simulink model "lock_srw_vB_windows"  (R2020a)
settings: Solver=FixedStepAuto  StartTime=0.0  StopTime=inf  RelTol=1e-3
model workspace (MAT data in the model file):
  PLC_IP_Address = 'localhost'
libraries: dspnetwork x29, simulink x2, utility x1
(part 1 of 2)
settings Model: SimulationMode=accelerator  EnablePacing=on  Creator=SueAnne  LastModifiedBy=jrsma
settings DataIOCC: ReturnWorkspaceOutputs=off
settings DebuggingCC: PregeneratedLibrarySubsystemCodeDiagnostic=none  ArithmeticOperatorsInVariantConditions=warning
settings SFSimCC: SimUseLocalCustomCode=off  CustomCodeUndefinedFunction=UseInterfaceOnly
settings RTWCC: PackageGeneratedCodeAndArtifacts=on  PackageName=Lock  RTWUseLocalCustomCode=off

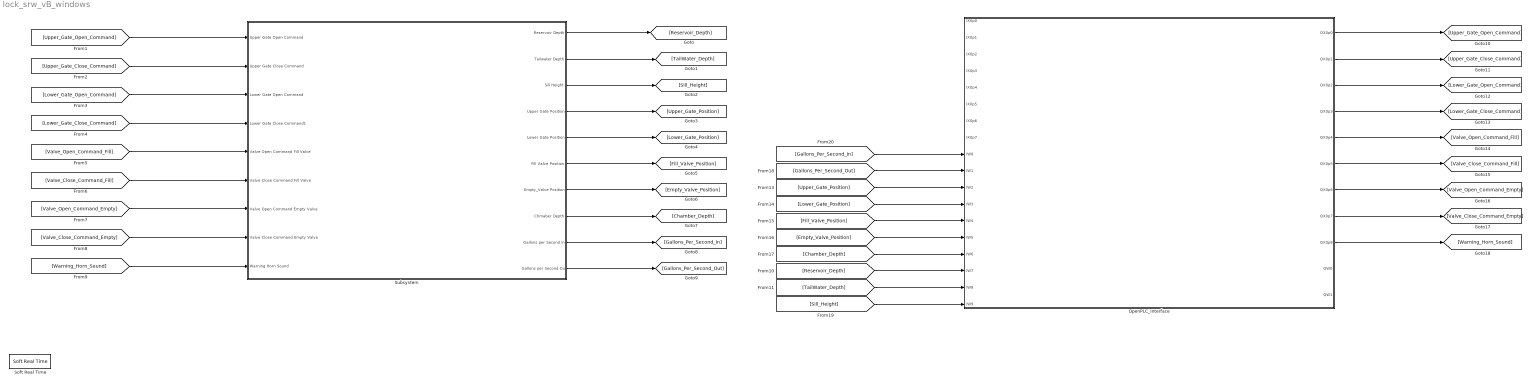
== system lock_srw_vB_windows ==
  OpenPLC_Interface : Subsystem
  Soft Real Time : utility/Soft Real Time  x=1
      settings: SourceProductName=Soft Real Time Lib
  Subsystem : Subsystem
  wires:
  [Upper_Gate_Open_Command] -> Subsystem/1(Upper Gate Open Command)
  [Upper_Gate_Close_Command] -> Subsystem/2(Upper Gate Close Command)
  [Lower_Gate_Open_Command] -> Subsystem/3(Lower Gate Open Command)
  [Lower_Gate_Close_Command] -> Subsystem/4(Lower Gate Close Command1)
  [Valve_Open_Command_Fill] -> Subsystem/5(Valve Open Command Fill Valve)
  [Valve_Close_Command_Fill] -> Subsystem/6(Valve Close Command Fill Valve)
  [Valve_Open_Command_Empty] -> Subsystem/7(Valve Open Command Empty Valve)
  [Valve_Close_Command_Empty] -> Subsystem/8(Valve Close Command Empty Valve)
  [Warning_Horn_Sound] -> Subsystem/9(Warning Horn Sound)
  Subsystem/1(Reservoir Depth) -> [Reservoir_Depth]
  Subsystem/2(Tailwater Depth) -> [TailWater_Depth]
  Subsystem/3(Sill Height) -> [Sill_Height]
  Subsystem/4(Upper Gate Position) -> [Upper_Gate_Position]
  Subsystem/5(Lower Gate Position) -> [Lower_Gate_Position]
  Subsystem/6(Fill Valve Position) -> [Fill_Valve_Position]
  Subsystem/7(Empty_Valve Position) -> [Empty_Valve_Position]
  Subsystem/8(Chmaber Depth) -> [Chamber_Depth]
  Subsystem/9(Gallons per Second In) -> [Gallons_Per_Second_In]
  Subsystem/10(Gallons per Second Ou) -> [Gallons_Per_Second_Out]
  [Sill_Height] -> OpenPLC_Interface/18(IW9)
  OpenPLC_Interface/1(QX0p0) -> [Upper_Gate_Open_Command]
  OpenPLC_Interface/2(QX0p1) -> [Upper_Gate_Close_Command]
  OpenPLC_Interface/3(QX0p2) -> [Lower_Gate_Open_Command]
  OpenPLC_Interface/4(QX0p3) -> [Lower_Gate_Close_Command]
  OpenPLC_Interface/5(QX0p4) -> [Valve_Open_Command_Fill]
  OpenPLC_Interface/6(QX0p5) -> [Valve_Close_Command_Fill]
  OpenPLC_Interface/7(QX0p6) -> [Valve_Open_Command_Empty]
  OpenPLC_Interface/8(QX0p7) -> [Valve_Close_Command_Empty]
  OpenPLC_Interface/9(QX0p8) -> [Warning_Horn_Sound]
  [Gallons_Per_Second_In] -> OpenPLC_Interface/9(IW0)
  [TailWater_Depth] -> OpenPLC_Interface/17(IW8)
  [Reservoir_Depth] -> OpenPLC_Interface/16(IW7)
  [Chamber_Depth] -> OpenPLC_Interface/15(IW6)
  [Empty_Valve_Position] -> OpenPLC_Interface/14(IW5)
  [Fill_Valve_Position] -> OpenPLC_Interface/13(IW4)
  [Lower_Gate_Position] -> OpenPLC_Interface/12(IW3)
  [Upper_Gate_Position] -> OpenPLC_Interface/11(IW2)
  [Gallons_Per_Second_Out] -> OpenPLC_Interface/10(IW1)

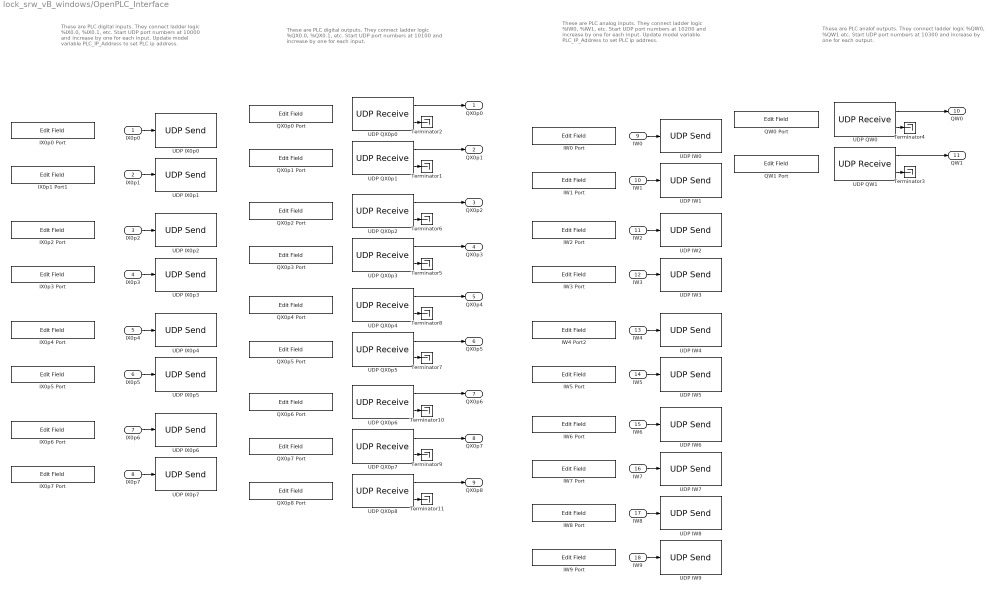
== system lock_srw_vB_windows/OpenPLC_Interface ==
  note: These are PLC digital inputs. They connect
      | ladder logic %IX0.0, %IX0.1, etc.
      |
      | Start UDP port numbers at 10000 and
      | increase by one for each input.
      |
      | Update model variable PLC_IP_Address
      | to set PLC ip address.
  note: These are PLC digital outputs. They connect
      | ladder logic %QX0.0, %QX0.1, etc.
      |
      | Start UDP port numbers at 10100 and increase
      | by one for each input.
  note: These are PLC analog inputs. They connect
      | ladder logic %IW0, %IW1, etc.
      |
      | Start UDP port numbers  at 10200 and
      | increase by one for each input.
      |
      | Update model variable PLC_IP_Address
      | to set PLC ip address.
  note: These are PLC analof outputs. They connect
      | ladder logic %QW0, %QW1 etc.
      |
      | Start UDP port numbers at 10300 and increase
      | by one for each output.
  "IX0p0 " : Inport
  IX0p1 : Inport  Port=2
  IX0p2 : Inport  Port=3
  IX0p3 : Inport  Port=4
  IX0p4 : Inport  Port=5
  IX0p5 : Inport  Port=6
  IX0p6 : Inport  Port=7
  IX0p7 : Inport  Port=8
  IW0 : Inport  Port=9
  IW1 : Inport  Port=10
  IW2 : Inport  Port=11
  IW3 : Inport  Port=12
  IW4 : Inport  Port=13
  IW5 : Inport  Port=14
  IW6 : Inport  Port=15
  IW7 : Inport  Port=16
  IW8 : Inport  Port=17
  IW9 : Inport  Port=18
  IW0 Port : EditField  LabelPosition=Hide  ShowInitialText=on  Alignment=Center
  IW1 Port : EditField  LabelPosition=Hide  ShowInitialText=on  Alignment=Center
  IW2 Port : EditField  LabelPosition=Hide  ShowInitialText=on  Alignment=Center
  IW3 Port : EditField  LabelPosition=Hide  ShowInitialText=on  Alignment=Center
  IW4 Port2 : EditField  LabelPosition=Hide  ShowInitialText=on  Alignment=Center
  IW5 Port : EditField  LabelPosition=Hide  ShowInitialText=on  Alignment=Center
  IW6 Port : EditField  LabelPosition=Hide  ShowInitialText=on  Alignment=Center
  IW7 Port : EditField  LabelPosition=Hide  ShowInitialText=on  Alignment=Center
  IW8 Port : EditField  LabelPosition=Hide  ShowInitialText=on  Alignment=Center
  IW9 Port : EditField  LabelPosition=Hide  ShowInitialText=on  Alignment=Center
  IX0p0 Port : EditField  LabelPosition=Hide  ShowInitialText=on  Alignment=Center
  IX0p1 Port1 : EditField  LabelPosition=Hide  ShowInitialText=on  Alignment=Center
  IX0p2 Port : EditField  LabelPosition=Hide  ShowInitialText=on  Alignment=Center
  IX0p3 Port : EditField  LabelPosition=Hide  ShowInitialText=on  Alignment=Center
  IX0p4 Port : EditField  LabelPosition=Hide  ShowInitialText=on  Alignment=Center
  IX0p5 Port : EditField  LabelPosition=Hide  ShowInitialText=on  Alignment=Center
  IX0p6 Port : EditField  LabelPosition=Hide  ShowInitialText=on  Alignment=Center
  IX0p7 Port : EditField  LabelPosition=Hide  ShowInitialText=on  Alignment=Center
  QW0 Port : EditField  LabelPosition=Hide  ShowInitialText=on  Alignment=Center
  QW1 Port : EditField  LabelPosition=Hide  ShowInitialText=on  Alignment=Center
  QX0p0 Port : EditField  LabelPosition=Hide  ShowInitialText=on  Alignment=Center
  QX0p1 Port : EditField  LabelPosition=Hide  ShowInitialText=on  Alignment=Center
  QX0p2 Port : EditField  LabelPosition=Hide  ShowInitialText=on  Alignment=Center
  QX0p3 Port : EditField  LabelPosition=Hide  ShowInitialText=on  Alignment=Center
  QX0p4 Port : EditField  LabelPosition=Hide  ShowInitialText=on  Alignment=Center
  QX0p5 Port : EditField  LabelPosition=Hide  ShowInitialText=on  Alignment=Center
  QX0p6 Port : EditField  LabelPosition=Hide  ShowInitialText=on  Alignment=Center
  QX0p7 Port : EditField  LabelPosition=Hide  ShowInitialText=on  Alignment=Center
  "QX0p8 Port " : EditField  LabelPosition=Hide  ShowInitialText=on  Alignment=Center
  Terminator{1..11} (11 alike) : Terminator
  UDP IW0 : dspnetwork/UDP Send  remoteURL='localhost'  remotePort=10200  localURL='255.255.255.255'  localPortSource=Automatically determine  localPort=-1  sendBufferSize=8192  sampletime=-1  blockPlatform=LINUX  separateLengthPort=0
  UDP IW1 : dspnetwork/UDP Send  remoteURL='localhost'  remotePort=10201  localURL='255.255.255.255'  localPortSource=Automatically determine  localPort=-1  sendBufferSize=8192  sampletime=-1  blockPlatform=LINUX  separateLengthPort=0
  UDP IW2 : dspnetwork/UDP Send  remoteURL='localhost'  remotePort=10202  localURL='255.255.255.255'  localPortSource=Automatically determine  localPort=-1  sendBufferSize=8192  sampletime=-1  blockPlatform=LINUX  separateLengthPort=0
  UDP IW3 : dspnetwork/UDP Send  remoteURL='localhost'  remotePort=10203  localURL='255.255.255.255'  localPortSource=Automatically determine  localPort=-1  sendBufferSize=8192  sampletime=-1  blockPlatform=LINUX  separateLengthPort=0
  UDP IW4 : dspnetwork/UDP Send  remoteURL='localhost'  remotePort=10204  localURL='255.255.255.255'  localPortSource=Automatically determine  localPort=-1  sendBufferSize=8192  sampletime=-1  blockPlatform=LINUX  separateLengthPort=0
  UDP IW5 : dspnetwork/UDP Send  remoteURL='localhost'  remotePort=10205  localURL='255.255.255.255'  localPortSource=Automatically determine  localPort=-1  sendBufferSize=8192  sampletime=-1  blockPlatform=LINUX  separateLengthPort=0
  UDP IW6 : dspnetwork/UDP Send  remoteURL='localhost'  remotePort=10206  localURL='255.255.255.255'  localPortSource=Automatically determine  localPort=-1  sendBufferSize=8192  sampletime=-1  blockPlatform=LINUX  separateLengthPort=0
  UDP IW7 : dspnetwork/UDP Send  remoteURL='localhost'  remotePort=10207  localURL='255.255.255.255'  localPortSource=Automatically determine  localPort=-1  sendBufferSize=8192  sampletime=-1  blockPlatform=LINUX  separateLengthPort=0
  UDP IW8 : dspnetwork/UDP Send  remoteURL='localhost'  remotePort=10208  localURL='255.255.255.255'  localPortSource=Automatically determine  localPort=-1  sendBufferSize=8192  sampletime=-1  blockPlatform=LINUX  separateLengthPort=0
  UDP IW9 : dspnetwork/UDP Send  remoteURL='localhost'  remotePort=10209  localURL='255.255.255.255'  localPortSource=Automatically determine  localPort=-1  sendBufferSize=8192  sampletime=-1  blockPlatform=LINUX  separateLengthPort=0
  UDP IX0p0 : dspnetwork/UDP Send  remoteURL='localhost'  remotePort=10000  localURL='255.255.255.255'  localPortSource=Automatically determine  localPort=-1  sendBufferSize=8192  sampletime=-1  blockPlatform=LINUX  separateLengthPort=0
  UDP IX0p1 : dspnetwork/UDP Send  remoteURL='localhost'  remotePort=10001  localURL='255.255.255.255'  localPortSource=Automatically determine  localPort=-1  sendBufferSize=8192  sampletime=-1  blockPlatform=LINUX  separateLengthPort=0
  UDP IX0p2 : dspnetwork/UDP Send  remoteURL='localhost'  remotePort=10002  localURL='255.255.255.255'  localPortSource=Automatically determine  localPort=-1  sendBufferSize=8192  sampletime=-1  blockPlatform=LINUX  separateLengthPort=0
  UDP IX0p3 : dspnetwork/UDP Send  remoteURL='localhost'  remotePort=10003  localURL='255.255.255.255'  localPortSource=Automatically determine  localPort=-1  sendBufferSize=8192  sampletime=-1  blockPlatform=LINUX  separateLengthPort=0
  UDP IX0p4 : dspnetwork/UDP Send  remoteURL='localhost'  remotePort=10004  localURL='255.255.255.255'  localPortSource=Automatically determine  localPort=-1  sendBufferSize=8192  sampletime=-1  blockPlatform=LINUX  separateLengthPort=0
  UDP IX0p5 : dspnetwork/UDP Send  remoteURL='localhost'  remotePort=10005  localURL='255.255.255.255'  localPortSource=Automatically determine  localPort=-1  sendBufferSize=8192  sampletime=-1  blockPlatform=LINUX  separateLengthPort=0
  UDP IX0p6 : dspnetwork/UDP Send  remoteURL='localhost'  remotePort=10006  localURL='255.255.255.255'  localPortSource=Automatically determine  localPort=-1  sendBufferSize=8192  sampletime=-1  blockPlatform=LINUX  separateLengthPort=0
  UDP IX0p7 : dspnetwork/UDP Send  remoteURL='localhost'  remotePort=10007  localURL='255.255.255.255'  localPortSource=Automatically determine  localPort=-1  sendBufferSize=8192  sampletime=-1  blockPlatform=LINUX  separateLengthPort=0
  UDP QW0 : dspnetwork/UDP Receive  localURL='0.0.0.0'  localPort=10300  remoteURL='0.0.0.0'  remotePort=-1  recvBufferSize=2  dims=1  signalDatatype=uint16  isComplex=off  isVarSize=off  showBlockingTime=on  blockingTime=0  sampletime=0.01  blockPlatform=LINUX
  UDP QW1 : dspnetwork/UDP Receive  localURL='0.0.0.0'  localPort=10301  remoteURL='0.0.0.0'  remotePort=-1  recvBufferSize=2  dims=1  signalDatatype=uint16  isComplex=off  isVarSize=off  showBlockingTime=on  blockingTime=0  sampletime=0.01  blockPlatform=LINUX
  UDP QX0p0 : dspnetwork/UDP Receive  localURL='0.0.0.0'  localPort=10100  remoteURL='0.0.0.0'  remotePort=-1  recvBufferSize=2  dims=1  signalDatatype=uint16  isComplex=off  isVarSize=off  showBlockingTime=on  blockingTime=0  sampletime=0.01  blockPlatform=LINUX
  UDP QX0p1 : dspnetwork/UDP Receive  localURL='0.0.0.0'  localPort=10101  remoteURL='0.0.0.0'  remotePort=-1  recvBufferSize=2  dims=1  signalDatatype=uint16  isComplex=off  isVarSize=off  showBlockingTime=on  blockingTime=0  sampletime=0.01  blockPlatform=LINUX
  UDP QX0p2 : dspnetwork/UDP Receive  localURL='0.0.0.0'  localPort=10102  remoteURL='0.0.0.0'  remotePort=-1  recvBufferSize=2  dims=1  signalDatatype=uint16  isComplex=off  isVarSize=off  showBlockingTime=on  blockingTime=0  sampletime=0.01  blockPlatform=LINUX
  UDP QX0p3 : dspnetwork/UDP Receive  localURL='0.0.0.0'  localPort=10103  remoteURL='0.0.0.0'  remotePort=-1  recvBufferSize=2  dims=1  signalDatatype=uint16  isComplex=off  isVarSize=off  showBlockingTime=on  blockingTime=0  sampletime=0.01  blockPlatform=LINUX
  UDP QX0p4 : dspnetwork/UDP Receive  localURL='0.0.0.0'  localPort=10104  remoteURL='0.0.0.0'  remotePort=-1  recvBufferSize=2  dims=1  signalDatatype=uint16  isComplex=off  isVarSize=off  showBlockingTime=on  blockingTime=0  sampletime=0.01  blockPlatform=LINUX
  UDP QX0p5 : dspnetwork/UDP Receive  localURL='0.0.0.0'  localPort=10105  remoteURL='0.0.0.0'  remotePort=-1  recvBufferSize=2  dims=1  signalDatatype=uint16  isComplex=off  isVarSize=off  showBlockingTime=on  blockingTime=0  sampletime=0.01  blockPlatform=LINUX
  UDP QX0p6 : dspnetwork/UDP Receive  localURL='0.0.0.0'  localPort=10106  remoteURL='0.0.0.0'  remotePort=-1  recvBufferSize=2  dims=1  signalDatatype=uint16  isComplex=off  isVarSize=off  showBlockingTime=on  blockingTime=0  sampletime=0.01  blockPlatform=LINUX
  UDP QX0p7 : dspnetwork/UDP Receive  localURL='0.0.0.0'  localPort=10107  remoteURL='0.0.0.0'  remotePort=-1  recvBufferSize=2  dims=1  signalDatatype=uint16  isComplex=off  isVarSize=off  showBlockingTime=on  blockingTime=0  sampletime=0.01  blockPlatform=LINUX
  UDP QX0p8 : dspnetwork/UDP Receive  localURL='0.0.0.0'  localPort=10108  remoteURL='0.0.0.0'  remotePort=-1  recvBufferSize=2  dims=1  signalDatatype=uint16  isComplex=off  isVarSize=off  showBlockingTime=on  blockingTime=0  sampletime=0.01  blockPlatform=LINUX
  QX0p0 : Outport
  QX0p1 : Outport  Port=2
  QX0p2 : Outport  Port=3
  QX0p3 : Outport  Port=4
  QX0p4 : Outport  Port=5
  QX0p5 : Outport  Port=6
  QX0p6 : Outport  Port=7
  QX0p7 : Outport  Port=8
  QX0p8 : Outport  Port=9
  QW0 : Outport  Port=10
  QW1 : Outport  Port=11
  wires:
  IX0p1/1 -> UDP IX0p1/1
  "IX0p0 "/1 -> UDP IX0p0/1
  UDP QX0p0/1 -> QX0p0/1
  UDP QX0p0/2 -> Terminator2/1
  UDP QX0p1/2 -> Terminator1/1
  UDP QX0p1/1 -> QX0p1/1
  IW1/1 -> UDP IW1/1
  IW0/1 -> UDP IW0/1
  UDP QW1/1 -> QW1/1
  UDP QW1/2 -> Terminator3/1
  UDP QW0/2 -> Terminator4/1
  UDP QW0/1 -> QW0/1
  IX0p2/1 -> UDP IX0p2/1
  IX0p3/1 -> UDP IX0p3/1
  IX0p7/1 -> UDP IX0p7/1
  IX0p6/1 -> UDP IX0p6/1
  IX0p4/1 -> UDP IX0p4/1
  IX0p5/1 -> UDP IX0p5/1
  UDP QX0p2/1 -> QX0p2/1
  UDP QX0p2/2 -> Terminator6/1
  UDP QX0p3/1 -> QX0p3/1
  UDP QX0p3/2 -> Terminator5/1
  UDP QX0p7/2 -> Terminator9/1
  UDP QX0p7/1 -> QX0p7/1
  UDP QX0p6/1 -> QX0p6/1
  UDP QX0p6/2 -> Terminator10/1
  UDP QX0p4/1 -> QX0p4/1
  UDP QX0p4/2 -> Terminator8/1
  UDP QX0p5/1 -> QX0p5/1
  UDP QX0p5/2 -> Terminator7/1
  IW3/1 -> UDP IW3/1
  IW2/1 -> UDP IW2/1
  IW7/1 -> UDP IW7/1
  IW5/1 -> UDP IW5/1
  IW4/1 -> UDP IW4/1
  IW6/1 -> UDP IW6/1
  IW9/1 -> UDP IW9/1
  IW8/1 -> UDP IW8/1
  UDP QX0p8/2 -> Terminator11/1
  UDP QX0p8/1 -> QX0p8/1

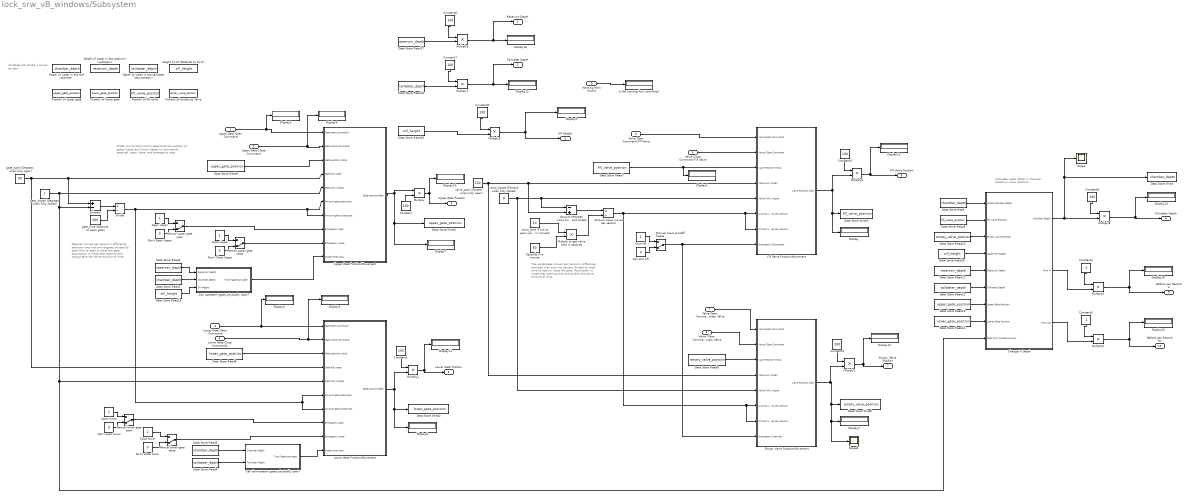
== system lock_srw_vB_windows/Subsystem ==
  note: These two function blocks determine the position of gates (upper and lower) based on commands received: open, close, and emergency stop.
  note: Variables are stored in boxes at right.
  note: Calculate water depth in chamber based on valve positions.
  note: Degrees moved per second is difference between max and min degrees divided by total time to open or close the gate. Assumption is made that opening and closing take the same amount of time.
  note: The percentage moved per second is difference between max and min percent divided by total time to open or close the gate. Assumption is made that opening and closing take the same amount of time.
  Upper Gate Open Command : Inport
  Upper Gate Close Command : Inport  Port=2
  Lower Gate Open Command : Inport  Port=3
  Lower Gate Close Command1 : Inport  Port=4
  Valve Open Command Fill Valve : Inport  Port=5
  Valve Close Command Fill Valve : Inport  Port=6
  Valve Open Command Empty Valve : Inport  Port=7
  Valve Close Command Empty Valve : Inport  Port=8
  Warning Horn Sound : Inport  Port=9
  Amount between valve fully open and closed : Sum  Inputs=-+  OutDataTypeStr=uint8
  Amount valve moves per second : Product  Inputs=*/  OutDataTypeStr=double
  Can downstream gates physically open? : Subsystem
  Can upstream gates physically open? : Subsystem
  Change in Depth : Subsystem
  Close Upper : Constant
  Close lower : Constant
  Constant{,1..3,6..9} (8 alike) : Constant  Value=100
  Constant4 : Constant  Value=.1
  Constant5 : Constant  Value=.1
  Data Store Read : DataStoreRead  DataStoreName=chamber_depth
  Data Store Read1 : DataStoreRead  Priority=0  DataStoreName=chamber_depth
  Data Store Read10 : DataStoreRead  DataStoreName=empty_valve_position
  Data Store Read11 : DataStoreRead  DataStoreName=reservoir_depth
  Data Store Read12 : DataStoreRead  DataStoreName=tailwater_depth
  Data Store Read13 : DataStoreRead  DataStoreName=upper_gate_position
  Data Store Read14 : DataStoreRead  DataStoreName=lower_gate_position
  Data Store Read15 : DataStoreRead  Priority=0  DataStoreName=sill_height
  Data Store Read16 : DataStoreRead  Priority=0  DataStoreName=sill_height
  Data Store Read17 : DataStoreRead  Priority=0  DataStoreName=reservoir_depth
  Data Store Read18 : DataStoreRead  Priority=0  DataStoreName=tailwater_depth
  Data Store Read19 : DataStoreRead  Priority=0  DataStoreName=sill_height
  Data Store Read2 : DataStoreRead  Priority=0  DataStoreName=reservoir_depth
  Data Store Read3 : DataStoreRead  DataStoreName=chamber_depth
  Data Store Read4 : DataStoreRead  DataStoreName=tailwater_depth
  Data Store Read5 : DataStoreRead  Priority=0  DataStoreName=upper_gate_position
  Data Store Read6 : DataStoreRead  Priority=0  DataStoreName=lower_gate_position
  Data Store Read7 : DataStoreRead  Priority=0  DataStoreName=fill_valve_position
  Data Store Read8 : DataStoreRead  Priority=0  DataStoreName=empty_valve_position
  Data Store Read9 : DataStoreRead  DataStoreName=fill_valve_position
  Data Store Write : DataStoreWrite  DataStoreName=chamber_depth
  Data Store Write1 : DataStoreWrite  Priority=9  DataStoreName=upper_gate_position
  Data Store Write2 : DataStoreWrite  Priority=9  DataStoreName=lower_gate_position
  Data Store Write3 : DataStoreWrite  Priority=9  DataStoreName=fill_valve_position
  Data Store Write4 : DataStoreWrite  Priority=9  DataStoreName=empty_valve_position
  Depth of water in the lock chamber : DataStoreMemory  DataStoreName=chamber_depth  ReadBeforeWriteMsg=warning  WriteAfterWriteMsg=warning  WriteAfterReadMsg=warning  InitialValue=42.5  ShowAdditionalParam=off
  Depth of water in the reservoir (upstream) : DataStoreMemory  DataStoreName=reservoir_depth  ReadBeforeWriteMsg=warning  WriteAfterWriteMsg=warning  WriteAfterReadMsg=warning  InitialValue=21  ShowAdditionalParam=off
  Depth of water in the tailwater (downstream) : DataStoreMemory  DataStoreName=tailwater_depth  ReadBeforeWriteMsg=warning  WriteAfterWriteMsg=warning  WriteAfterReadMsg=warning  InitialValue=21  ShowAdditionalParam=off
  Display{,1..16,18..19} (19 alike) : Display
  Divide : Product  Inputs=*/  OutDataTypeStr=double
  Don't Close Upper : Constant  Value=0
  Don't Open Upper : Constant  Value=0
  Don't close lower : Constant  Value=0
  Don't open lower : Constant  Value=0
  Empty Valve Position/Movement : Subsystem
  Fill Valve Position/Movement : Subsystem
  Height of sill (Defaults to 21.5') : DataStoreMemory  DataStoreName=sill_height  ReadBeforeWriteMsg=warning  WriteAfterWriteMsg=warning  WriteAfterReadMsg=warning  InitialValue=21.5  ShowAdditionalParam=off
  Is the warning horn sounding? : Display
  Lower Gate Position/Movement : Subsystem
  Manual lower gate close : ManualSwitch  CurrentSetting=0
  Manual lower gate open : ManualSwitch  CurrentSetting=0
  Manual upper gate close : ManualSwitch  CurrentSetting=0
  Manual upper gate open : ManualSwitch  CurrentSetting=0
  Manual valve shutoff/ freeze : ManualSwitch  CurrentSetting=0
  Multiply{,1..9} (10 alike) : Product
  Multiply to get valve time in seconds : Product  OutDataTypeStr=uint16
  Not shut off : Constant  Value=0  OutDataTypeStr=boolean
  Open Upper : Constant
  Open lower : Constant
  Position of emptying valve : DataStoreMemory  DataStoreName=empty_valve_position  ReadBeforeWriteMsg=warning  WriteAfterWriteMsg=warning  WriteAfterReadMsg=warning  ShowAdditionalParam=off
  Position of fill valve : DataStoreMemory  DataStoreName=fill_valve_position  ReadBeforeWriteMsg=warning  WriteAfterWriteMsg=warning  WriteAfterReadMsg=warning  ShowAdditionalParam=off  OutMin=0  OutMax=100  OutDataTypeStr=double
  Position of lower gate : DataStoreMemory  DataStoreName=lower_gate_position  ReadBeforeWriteMsg=warning  WriteAfterWriteMsg=warning  WriteAfterReadMsg=warning  InitialValue=7  ShowAdditionalParam=off
  Position of upper gate : DataStoreMemory  DataStoreName=upper_gate_position  ReadBeforeWriteMsg=warning  WriteAfterWriteMsg=warning  WriteAfterReadMsg=warning  InitialValue=7  ShowAdditionalParam=off
  Scope : Scope
  Scope1 : Scope
  Seconds in a minute : Constant  Value=60  OutDataTypeStr=uint8
  Shut off : Constant  OutDataTypeStr=boolean
  Subtract : Sum  Inputs=+-
  Upper Gate Position/Movement : Subsystem
  gate_closed (Degrees when fully closed) : Constant  Value=7
  gate_open (Degrees when fully open) : Constant  Value=90
  gate_time (Seconds to open gate) : Constant  Value=300
  valve_closed (Percent when fully closed) : Constant  Value=0  OutDataTypeStr=uint8
  valve_open (Percent when fully open) : Constant  Value=100  OutDataTypeStr=uint8
  "valve_time (Time to open valve, in minutes)" : Constant  Value=10  OutDataTypeStr=uint8
  Reservoir Depth : Outport
  Tailwater Depth : Outport  Port=2
  Sill Height : Outport  Port=3
  Upper Gate Position : Outport  Port=4
  Lower Gate Position : Outport  Port=5
  Fill Valve Position : Outport  Port=6
  Empty_Valve Position : Outport  Port=7
  Chmaber Depth : Outport  Port=8
  Gallons per Second In : Outport  Port=9
  Gallons per Second Ou : Outport  Port=10
  wires:
  Divide/1 -> Lower Gate Position/Movement/7(Amount gate closes/sec), Lower Gate Position/Movement/6(Amount gate opens/sec), Upper Gate Position/Movement/7(Amount gate closes/sec), Upper Gate Position/Movement/6(Amount gate opens/sec)
  Empty Valve Position/Movement/1(Valve Position After) -> Multiply2/2, Scope1/1, Display2/1, Data Store Write4/1
  Data Store Read1/1 -> Can upstream gates physically open?/2(Chamber Depth)
  Amount between valve fully open and closed/1 -> Amount valve moves per second/1
  Data Store Read3/1 -> Can downstream gates physically open?/1(Chamber Depth)
  Upper Gate Position/Movement/1(Gate position after) -> Multiply/1, Display7/1, Data Store Write1/1
  Constant3/1 -> Multiply3/1
  Fill Valve Position/Movement/1(Valve Position After) -> Multiply3/2, Data Store Write3/1, Display/1
  gate_closed (Degrees when fully closed)/1 -> Change in Depth/9(Gate Fully Closed Amount), Lower Gate Position/Movement/5(Gate fully closed), Subtract/2, Upper Gate Position/Movement/5(Gate fully closed)
  Lower Gate Position/Movement/1(Gate position after) -> Multiply1/2, Data Store Write2/1, Display8/1
  Manual lower gate open/1 -> Lower Gate Position/Movement/8(Emergency open)
  Can upstream gates physically open?/1(True if gate can open) -> Upper Gate Position/Movement/10(Water level okay)
  gate_time (Seconds to open gate)/1 -> Divide/2
  Can downstream gates physically open?/1(True if gate can open) -> Lower Gate Position/Movement/10(Water level okay)
  Amount valve moves per second/1 -> Fill Valve Position/Movement/7(Amount valve closes per second), Fill Valve Position/Movement/6(Amount valve opens per second), Empty Valve Position/Movement/7(Amount valve closes per second), Empty Valve Position/Movement/6(Amount valve opens per second)
  Data Store Read4/1 -> Can downstream gates physically open?/2(Tailwater Depth)
  Data Store Read6/1 -> Lower Gate Position/Movement/3(Gate position initial)
  Shut off/1 -> Manual valve shutoff/ freeze/1
  valve_closed (Percent when fully closed)/1 -> Fill Valve Position/Movement/5(Valve Fully Closed), Amount between valve fully open and closed/1, Empty Valve Position/Movement/5(Valve Fully Closed)
  Open lower/1 -> Manual lower gate open/1
  Data Store Read/1 -> Change in Depth/1(Initial Chamber Depth)
  Constant2/1 -> Multiply2/1
  Change in Depth/1(Chamber Depth) -> Multiply8/2, Scope/1, Data Store Write/1
  Don't Close Upper/1 -> Manual upper gate close/2
  Data Store Read11/1 -> Change in Depth/5(Reservoir Depth)
  Data Store Read9/1 -> Change in Depth/2(Fill Valve Position)
  Data Store Read17/1 -> Multiply6/2
  Data Store Read13/1 -> Change in Depth/7(Upper Gate Position)
  Data Store Read15/1 -> Can upstream gates physically open?/3(Sill Height)
  Change in Depth/3(Flow out) -> Multiply5/2
  gate_open (Degrees when fully open)/1 -> Lower Gate Position/Movement/4(Gate fully open), Subtract/1, Upper Gate Position/Movement/4(Gate fully open)
  Upper Gate Close Command/1 -> Upper Gate Position/Movement/2(Gate close command), Display4/1
  valve_open (Percent when fully open)/1 -> Amount between valve fully open and closed/2, Fill Valve Position/Movement/4(Valve Fully Open), Empty Valve Position/Movement/4(Valve Fully Open)
  Data Store Read7/1 -> Display1/1, Fill Valve Position/Movement/3(Valve Position Initial)
  Close lower/1 -> Manual lower gate close/1
  Manual valve shutoff/ freeze/1 -> Fill Valve Position/Movement/8(Emergency Disconnect), Empty Valve Position/Movement/8(Emergency Override)
  Constant/1 -> Multiply/2
  Data Store Read2/1 -> Can upstream gates physically open?/1(Reservoir Depth)
  Constant1/1 -> Multiply1/1
  Manual upper gate close/1 -> Upper Gate Position/Movement/9(Emergency close)
  Data Store Read16/1 -> Change in Depth/4(Upper Sill Height)
  Lower Gate Close Command1/1 -> Lower Gate Position/Movement/2(Gate close command), Display6/1
  Close Upper/1 -> Manual upper gate close/1
  Don't close lower/1 -> Manual lower gate close/2
  Not shut off/1 -> Manual valve shutoff/ freeze/2
  Multiply5/1 -> Gallons per Second Ou/1, Display19/1
  Data Store Read12/1 -> Change in Depth/6(Tailwater Depth)
  Data Store Read8/1 -> Empty Valve Position/Movement/3(Valve Position Initial)
  Change in Depth/2(Flow in) -> Multiply4/2
  Constant4/1 -> Multiply4/1
  Warning Horn Sound/1 -> Is the warning horn sounding?/1
  Multiply/1 -> Upper Gate Position/1, Display10/1
  Data Store Read5/1 -> Upper Gate Position/Movement/3(Gate position initial)
  Open Upper/1 -> Manual upper gate open/1
  Constant6/1 -> Multiply6/1
  Multiply to get valve time in seconds/1 -> Amount valve moves per second/2
  Don't open lower/1 -> Manual lower gate open/2
  Multiply7/1 -> Tailwater Depth/1, Display15/1
  Don't Open Upper/1 -> Manual upper gate open/2
  Seconds in a minute/1 -> Multiply to get valve time in seconds/2
  Constant7/1 -> Multiply7/1
  Manual upper gate open/1 -> Upper Gate Position/Movement/8(Emergency open)
  Data Store Read18/1 -> Multiply7/2
  Constant8/1 -> Multiply8/1
  Data Store Read10/1 -> Change in Depth/3(Empty Valve Position)
  Manual lower gate close/1 -> Lower Gate Position/Movement/9(Emergency close)
  Constant5/1 -> Multiply5/1
  Data Store Read14/1 -> Change in Depth/8(Lower Gate Position)
  Lower Gate Open Command/1 -> Lower Gate Position/Movement/1(Gate open command), Display5/1
  "valve_time (Time to open valve, in minutes)"/1 -> Multiply to get valve time in seconds/1
  Subtract/1 -> Divide/1
  Upper Gate Open Command/1 -> Display3/1, Upper Gate Position/Movement/1(Gate open command)
  Valve Open Command Fill Valve/1 -> Fill Valve Position/Movement/1(Valve Open Command)
  Valve Close Command Fill Valve/1 -> Fill Valve Position/Movement/2(Valve Close Command)
  Valve Open Command Empty Valve/1 -> Empty Valve Position/Movement/1(Valve Open Command)
  Valve Close Command Empty Valve/1 -> Empty Valve Position/Movement/2(Valve Close Command)
  Multiply6/1 -> Reservoir Depth/1, Display16/1
  Multiply1/1 -> Lower Gate Position/1, Display11/1
  Multiply3/1 -> Fill Valve Position/1, Display13/1
  Multiply2/1 -> Empty_Valve Position/1, Display12/1
  Multiply8/1 -> Chmaber Depth/1, Display14/1
  Multiply4/1 -> Gallons per Second In/1, Display18/1
  Data Store Read19/1 -> Multiply9/2
  Multiply9/1 -> Display9/1, Sill Height/1
  Constant9/1 -> Multiply9/1

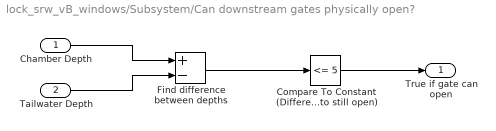
== system lock_srw_vB_windows/Subsystem/Can downstream gates physically open? ==
  Chamber Depth : Inport
  Tailwater Depth : Inport  Port=2
  Compare To Constant (Difference allowed between depths for gate to still open) : simulink/Logic and Bit Operations/Compare To Constant  relop=<=  const=5  OutDataTypeStr=boolean
  Find difference between depths : Sum  Inputs=+-
  True if gate can open : Outport  VectorParamsAs1DForOutWhenUnconnected=off
  wires:
  Chamber Depth/1 -> Find difference between depths/1
  Tailwater Depth/1 -> Find difference between depths/2
  Compare To Constant (Difference allowed between depths for gate to still open)/1 -> True if gate can open/1
  Find difference between depths/1 -> Compare To Constant (Difference allowed between depths for gate to still open)/1

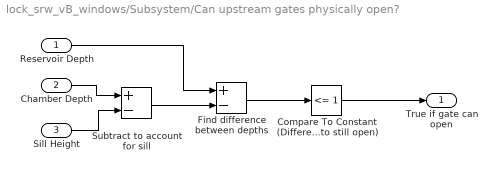
== system lock_srw_vB_windows/Subsystem/Can upstream gates physically open? ==
  Reservoir Depth : Inport
  Chamber Depth : Inport  Port=2
  Sill Height : Inport  Port=3
  Compare To Constant (Difference allowed between depths for gate to still open) : simulink/Logic and Bit Operations/Compare To Constant  relop=<=  const=1  OutDataTypeStr=boolean
  Find difference between depths : Sum  Inputs=+-
  Subtract to account for sill : Sum  Inputs=+-
  True if gate can open : Outport  VectorParamsAs1DForOutWhenUnconnected=off
  wires:
  Compare To Constant (Difference allowed between depths for gate to still open)/1 -> True if gate can open/1
  Find difference between depths/1 -> Compare To Constant (Difference allowed between depths for gate to still open)/1
  Subtract to account for sill/1 -> Find difference between depths/2
  Chamber Depth/1 -> Subtract to account for sill/1
  Sill Height/1 -> Subtract to account for sill/2
  Reservoir Depth/1 -> Find difference between depths/1

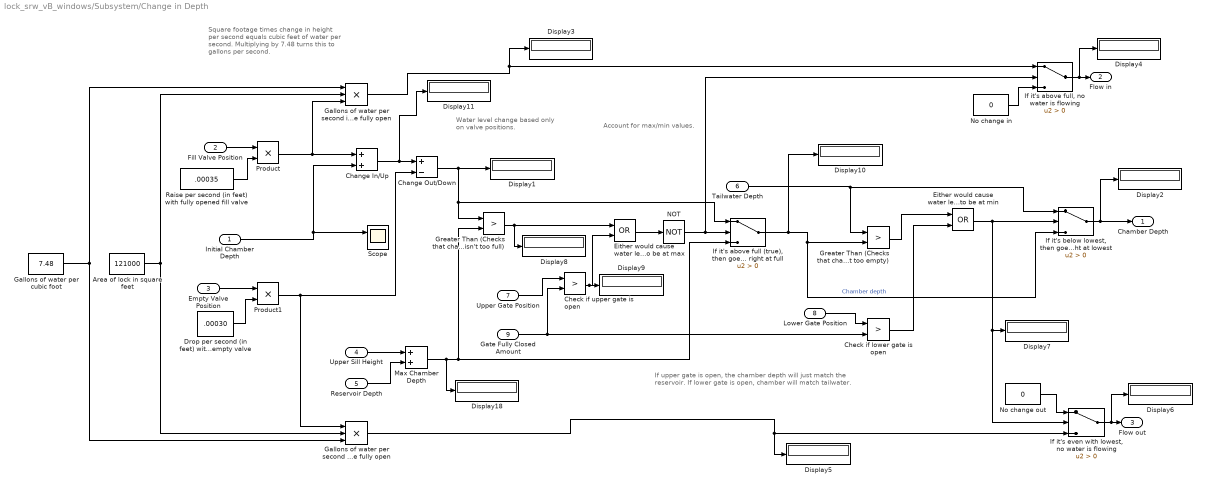
== system lock_srw_vB_windows/Subsystem/Change in Depth ==
  note: If upper gate is open, the chamber depth will just match the reservoir. If lower gate is open, chamber will match tailwater.
  note: Water level change based only on valve positions.
  note: Account for max/min values.
  note: Square footage times change in height per second equals cubic feet of water per second. Multiplying by 7.48 turns this to gallons per second.
  Initial Chamber Depth : Inport
  Fill Valve Position : Inport  Port=2
  Empty Valve Position : Inport  Port=3
  Upper Sill Height : Inport  Port=4
  Reservoir Depth : Inport  Port=5
  Tailwater Depth : Inport  Port=6
  Upper Gate Position : Inport  Port=7
  Lower Gate Position : Inport  Port=8
  Gate Fully Closed Amount : Inport  Port=9
  Area of lock in square feet : Constant  Value=121000  OutDataTypeStr=double
  Change Out/Down : Sum  Inputs=+-
  Change In/Up : Sum
  Check if lower gate is open : RelationalOperator  Operator=>  OutDataTypeStr=boolean  RndMeth=Simplest
  Check if upper gate is open : RelationalOperator  Operator=>  OutDataTypeStr=boolean  RndMeth=Simplest
  Display{1..11,18} (12 alike) : Display
  Drop per second (in feet) with fully opened empty valve : Constant  Value=.00030  OutDataTypeStr=double
  Either would cause water level to be at max : Logic  Operator=OR  AllPortsSameDT=off  OutDataTypeStr=boolean
  Either would cause water level to be at min : Logic  Operator=OR  AllPortsSameDT=off  OutDataTypeStr=boolean
  Gallons of water per cubic foot : Constant  Value=7.48  OutDataTypeStr=double
  "Gallons of water per second in, when fill valve fully open" : Product  Inputs=3
  "Gallons of water per second out, when empty valve fully open" : Product  Inputs=3
  Greater Than (Checks that chamber isn't too empty) : RelationalOperator  Operator=>  OutDataTypeStr=boolean  RndMeth=Simplest
  Greater Than (Checks that chamber isn't too full) : RelationalOperator  Operator=>  OutDataTypeStr=boolean  RndMeth=Simplest
  "If it's above full (true), then goes back to being right at full" : Switch  Criteria=u2 > Threshold
  "If it's above full, no water is flowing" : Switch  Criteria=u2 > Threshold
  "If it's below lowest, then goes back to being right at lowest" : Switch  Criteria=u2 > Threshold
  "If it's even with lowest, no water is flowing" : Switch  Criteria=u2 > Threshold
  Max Chamber Depth : Sum
  NOT : Logic  Operator=NOT  IconShape=distinctive  AllPortsSameDT=off  OutDataTypeStr=boolean
  No change in : Constant  Value=0  OutDataTypeStr=double
  No change out : Constant  Value=0  OutDataTypeStr=double
  Product : Product
  Product1 : Product
  Raise per second (in feet) with fully opened fill valve : Constant  Value=.00035  OutDataTypeStr=double
  Scope : Scope  NumInputPorts=2
  Chamber Depth : Outport  VectorParamsAs1DForOutWhenUnconnected=off
  Flow in : Outport  Port=2  VectorParamsAs1DForOutWhenUnconnected=off
  Flow out : Outport  Port=3  VectorParamsAs1DForOutWhenUnconnected=off
  wires:
  Fill Valve Position/1 -> Product/1
  Product/1 -> "Gallons of water per second in, when fill valve fully open"/3, Change In/Up/1
  Change In/Up/1 -> Display11/1, Change Out/Down/1
  Empty Valve Position/1 -> Product1/1
  Product1/1 -> "Gallons of water per second out, when empty valve fully open"/1, Change Out/Down/2
  Upper Sill Height/1 -> Max Chamber Depth/1
  Reservoir Depth/1 -> Max Chamber Depth/2
  Max Chamber Depth/1 -> Display18/1, Greater Than (Checks that chamber isn't too full)/2, "If it's above full (true), then goes back to being right at full"/3
  Change Out/Down/1 -> "If it's above full (true), then goes back to being right at full"/1, Greater Than (Checks that chamber isn't too full)/1, Display1/1
  "If it's above full (true), then goes back to being right at full"/1 -> Display10/1, Greater Than (Checks that chamber isn't too empty)/2, "If it's below lowest, then goes back to being right at lowest"/3  "Chamber depth"
  Greater Than (Checks that chamber isn't too full)/1 -> Either would cause water level to be at max/1, Display8/1
  Upper Gate Position/1 -> Check if upper gate is open/1
  Gate Fully Closed Amount/1 -> Check if upper gate is open/2, Check if lower gate is open/2
  Greater Than (Checks that chamber isn't too empty)/1 -> Either would cause water level to be at min/1
  Either would cause water level to be at min/1 -> Display7/1, "If it's even with lowest, no water is flowing"/2, "If it's below lowest, then goes back to being right at lowest"/2
  Lower Gate Position/1 -> Check if lower gate is open/1
  "If it's below lowest, then goes back to being right at lowest"/1 -> Display2/1, Chamber Depth/1
  Check if upper gate is open/1 -> Either would cause water level to be at max/2, Display9/1
  Gallons of water per cubic foot/1 -> "Gallons of water per second in, when fill valve fully open"/1, "Gallons of water per second out, when empty valve fully open"/3
  Initial Chamber Depth/1 -> Scope/1, Change In/Up/2
  Drop per second (in feet) with fully opened empty valve/1 -> Product1/2
  Raise per second (in feet) with fully opened fill valve/1 -> Product/2
  Area of lock in square feet/1 -> "Gallons of water per second out, when empty valve fully open"/2, "Gallons of water per second in, when fill valve fully open"/2
  "Gallons of water per second in, when fill valve fully open"/1 -> "If it's above full, no water is flowing"/1, Display3/1
  "If it's above full, no water is flowing"/1 -> Display4/1, Flow in/1
  No change in/1 -> "If it's above full, no water is flowing"/3
  Check if lower gate is open/1 -> Either would cause water level to be at min/2
  "If it's even with lowest, no water is flowing"/1 -> Flow out/1, Display6/1
  "Gallons of water per second out, when empty valve fully open"/1 -> Display5/1, "If it's even with lowest, no water is flowing"/3
  Tailwater Depth/1 -> Greater Than (Checks that chamber isn't too empty)/1, "If it's below lowest, then goes back to being right at lowest"/1
  NOT/1 -> "If it's above full, no water is flowing"/2, "If it's above full (true), then goes back to being right at full"/2
  Either would cause water level to be at max/1 -> NOT/1
  No change out/1 -> "If it's even with lowest, no water is flowing"/1

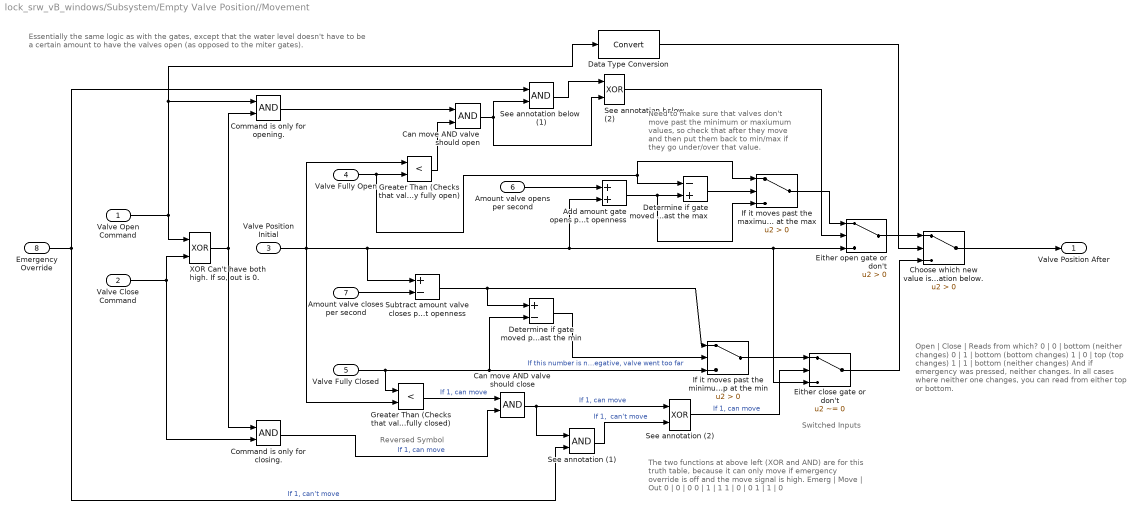
== system lock_srw_vB_windows/Subsystem/Empty Valve Position//Movement ==
  note: Switched Inputs
  note: Reversed Symbol
  note: Essentially the same logic as with the gates, except that the water level doesn't have to be a certain amount to have the valves open (as opposed to the miter gates).
  note: Open	|	Close	|	Reads from which?
      | 0		|	0		|	bottom (neither changes)
      | 0		|	1		|	bottom (bottom changes)
      | 1		|	0		|	top (top changes)
      | 1		|	1		|	bottom (neither changes)
      |
      | And if emergency was pressed, neither changes.  In all cases where neither one changes, you can read from either top or bottom.
  note: The two functions at above left (XOR and AND) are for this truth table, because it can only move if emergency override is off and the move signal is high.
      |
      | Emerg	|	Move	| Out
      | 0		|	0		|	0
      | 0		|	1		|	1
      | 1		|	0		|	0
      | 1		|	1		|	0
  note: Need to make sure that valves don't move past the minimum or maxiumum values, so check that after they move and then put them back to min/max if they go under/over that value.
  Valve Open Command : Inport
  Valve Close Command : Inport  Port=2
  Valve Position Initial : Inport  Port=3
  Valve Fully Open : Inport  Port=4
  Valve Fully Closed : Inport  Port=5
  Amount valve opens per second : Inport  Port=6
  Amount valve closes per second : Inport  Port=7
  Emergency Override : Inport  Port=8
  Add amount gate opens per second to current openness : Sum
  Can move AND valve should close : Logic  AllPortsSameDT=off  OutDataTypeStr=boolean
  Can move AND valve should open : Logic  AllPortsSameDT=off  OutDataTypeStr=boolean
  "Choose which new value is correct, based upon the open command. See annotation below." : Switch  Criteria=u2 > Threshold
  Command is only for closing. : Logic  AllPortsSameDT=off  OutDataTypeStr=boolean
  Command is only for opening. : Logic  AllPortsSameDT=off  OutDataTypeStr=boolean
  Data Type Conversion : DataTypeConversion
  Determine if gate moved past the max : Sum  Inputs=-+
  Determine if gate moved past the min : Sum  Inputs=+-
  Either close gate or don't : Switch  Criteria=u2 ~= 0  RndMeth=Simplest
  Either open gate or don't : Switch  Criteria=u2 > Threshold
  Greater Than (Checks that valve isn't already fully closed) : RelationalOperator  Operator=<  OutDataTypeStr=boolean  RndMeth=Simplest
  Greater Than (Checks that valve isn't already fully open) : RelationalOperator  Operator=<  OutDataTypeStr=boolean  RndMeth=Simplest
  "If it moves past the maximum, it will stop at the max" : Switch  Criteria=u2 > Threshold
  "If it moves past the minimum, it will stop at the min" : Switch  Criteria=u2 > Threshold
  See annotation below  (1) : Logic  AllPortsSameDT=off  OutDataTypeStr=boolean
  See annotation below (2) : Logic  Operator=XOR  IconShape=distinctive  AllPortsSameDT=off  OutDataTypeStr=boolean
  See annotation (1) : Logic  AllPortsSameDT=off  OutDataTypeStr=boolean
  See annotation (2) : Logic  Operator=XOR  IconShape=distinctive  AllPortsSameDT=off  OutDataTypeStr=boolean
  Subtract amount valve closes per second from current openness : Sum  Inputs=+-
  "XOR Can't have both high. If so, out is 0." : Logic  Operator=XOR  IconShape=distinctive  AllPortsSameDT=off  OutDataTypeStr=boolean
  Valve Position After : Outport  VectorParamsAs1DForOutWhenUnconnected=off
  wires:
  Command is only for opening./1 -> Can move AND valve should open/1
  Greater Than (Checks that valve isn't already fully open)/1 -> Can move AND valve should open/2
  Either open gate or don't/1 -> "Choose which new value is correct, based upon the open command. See annotation below."/1
  See annotation (1)/1 -> See annotation (2)/2  "If 1,  can't move"
  Valve Open Command/1 -> Data Type Conversion/1, Command is only for opening./1, "XOR Can't have both high. If so, out is 0."/1
  Valve Fully Open/1 -> Determine if gate moved past the max/1, "If it moves past the maximum, it will stop at the max"/1, Greater Than (Checks that valve isn't already fully open)/2
  "If it moves past the maximum, it will stop at the max"/1 -> Either open gate or don't/1
  Subtract amount valve closes per second from current openness/1 -> "If it moves past the minimum, it will stop at the min"/1, Determine if gate moved past the min/1
  Can move AND valve should open/1 -> See annotation below (2)/2, See annotation below  (1)/2
  Amount valve closes per second/1 -> Subtract amount valve closes per second from current openness/2
  See annotation below  (1)/1 -> See annotation below (2)/1
  Valve Position Initial/1 -> Greater Than (Checks that valve isn't already fully open)/1, Either close gate or don't/3, Either open gate or don't/3, Add amount gate opens per second to current openness/2, Subtract amount valve closes per second from current openness/1, Greater Than (Checks that valve isn't already fully closed)/2
  Either close gate or don't/1 -> "Choose which new value is correct, based upon the open command. See annotation below."/3
  Emergency Override/1 -> See annotation below  (1)/1, See annotation (1)/2  "If 1, can't move"
  See annotation below (2)/1 -> Either open gate or don't/2
  Valve Close Command/1 -> Command is only for closing./2, "XOR Can't have both high. If so, out is 0."/2
  Command is only for closing./1 -> Can move AND valve should close/2  "If 1, can move"
  See annotation (2)/1 -> Either close gate or don't/2  "If 1, can move"
  Can move AND valve should close/1 -> See annotation (2)/1, See annotation (1)/1  "If 1, can move"
  Add amount gate opens per second to current openness/1 -> Determine if gate moved past the max/2, "If it moves past the maximum, it will stop at the max"/3
  Determine if gate moved past the min/1 -> "If it moves past the minimum, it will stop at the min"/2  "If this number is negative, valve went too far"
  Greater Than (Checks that valve isn't already fully closed)/1 -> Can move AND valve should close/1  "If 1, can move"
  Valve Fully Closed/1 -> "If it moves past the minimum, it will stop at the min"/3, Determine if gate moved past the min/2, Greater Than (Checks that valve isn't already fully closed)/1
  Determine if gate moved past the max/1 -> "If it moves past the maximum, it will stop at the max"/2
  "XOR Can't have both high. If so, out is 0."/1 -> Command is only for closing./1, Command is only for opening./2
  Amount valve opens per second/1 -> Add amount gate opens per second to current openness/1
  "Choose which new value is correct, based upon the open command. See annotation below."/1 -> Valve Position After/1
  Data Type Conversion/1 -> "Choose which new value is correct, based upon the open command. See annotation below."/2
  "If it moves past the minimum, it will stop at the min"/1 -> Either close gate or don't/1
